simulink model "PI_current_no_modulatiob"  (R2018b)
settings: Solver=ode45  StartTime=0.0  StopTime=10  MaxStep=1e-3  RelTol=1e-6
values from neighbouring files (symbols this model uses):
  In = 189    [Motor_parameters_project.m]
  J = 0.0151    [Motor_parameters_project.m]
  Lm = 0.38e-3    (= 0.00038)    [Motor_parameters_project.m]
  Lr = Lm + Ldr    (= 0.00041116)    [Motor_parameters_project.m]
  Ls = Lm + Lds    (= 0.00041116)    [Motor_parameters_project.m]
  Omegae = 2*pi*fn    (= 364.424747816)    [Motor_parameters_project.m]
  p = 2.0    (= 2)    [Motor_parameters_project.m]
  Rr = 2.69e-3    (= 0.00269)    [Motor_parameters_project.m]
  Rs = 2.5e-3    (= 0.0025)    [Motor_parameters_project.m]
  Un = 24/sqrt(3)    [Motor_parameters_project.m]
undefined symbols (not defined in the file or in its folder): landa_r
settings Model: Creator=estef  LastModifiedBy=estef

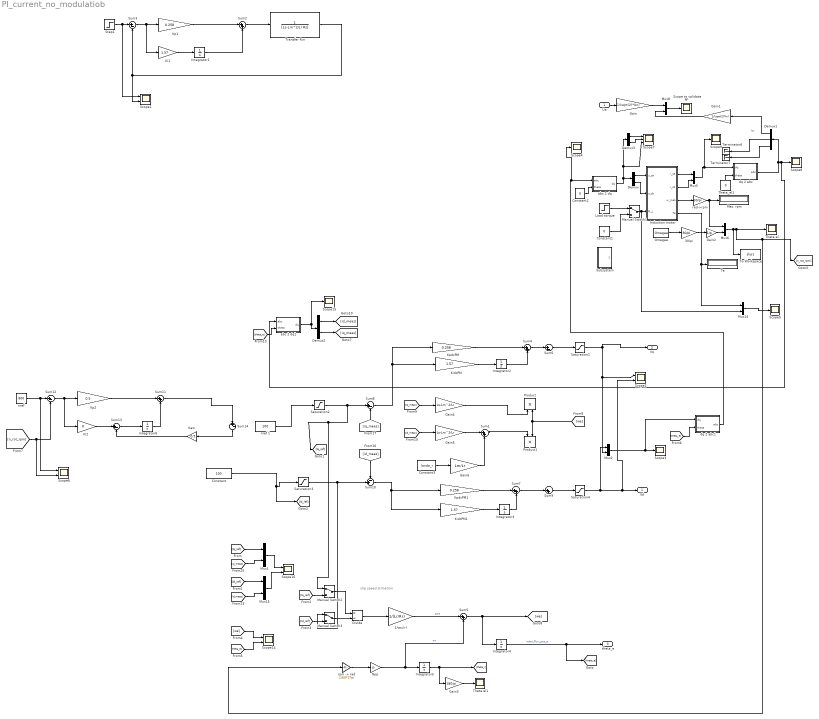
== system PI_current_no_modulatiob ==
  note: Ia
  note: slip speed stimation
  Ua : Inport
  1/tau(r) : Gain  Gain=1/(Lr/Rr)
  30/pi : Gain  Gain=30/pi
  Constant : Constant  Value=100
  Constant1 : Constant  Value=0
  Constant2 : Constant  Value=0
  Constant3 : Constant  Value=landa_r
  Demux : Demux  Outputs=2
  Demux1 : Demux  Outputs=3
  Demux2 : Demux  Outputs=2
  Demux3 : Demux  Outputs=2
  Divide : Product  Inputs=*/
  Gain : Gain  Gain=1/(sqrt(2)*Un)
  Gain1 : Gain  Gain=1/(sqrt(2)*In)
  Gain2 : Gain  Gain=1/p
  Gain3 : Gain  Gain=180/pi
  Gain4 : Gain  Gain=Ls-Lm^2/Lr
  Gain5 : Gain  Gain=Ls-Lm^2/Lr
  Gain6 : Gain  Gain=Lm/Lr
  Induction motor : Subsystem
  Integrator{1..6} (6 alike) : Integrator
  Kaw : Gain  Gain=0.5
  Ki1 : Gain  Gain=1.57
  Ki2 : Gain  Gain=0
  KidcPM : Gain  Gain=1.57
  KidcPM1 : Gain  Gain=1.57
  Kp1 : Gain  Gain=0.258
  Kp2 : Gain  Gain=0.5
  KpdcPM : Gain  Gain=0.258
  KpdcPM1 : Gain  Gain=0.258
  Load torque : Step  Time=0.9  After=5  SampleTime=0
  Manual Switch1 : ManualSwitch
  Manual Switch2 : ManualSwitch
  Manual Switch3 : ManualSwitch
  Mec. rpm : Display
  Mux{1..2,5..6,8,14..15} (7 alike) : Mux  Inputs=2
  Npp : Gain  Gain=p  SaturateOnIntegerOverflow=on  OutDataTypeStr=Inherit: Same as input  ParamDataTypeStr=Inherit: Same as input
  Omegae : Constant  Value=Omegae
  Product : Product  SaturateOnIntegerOverflow=on  InputSameDT=on  OutDataTypeStr=Inherit: Same as first input
  Product1 : Product  SaturateOnIntegerOverflow=on  InputSameDT=on  OutDataTypeStr=Inherit: Same as first input
  Saturation1 : Saturate  UpperLimit=Un*sqrt(2)  LowerLimit=-Un*sqrt(2)
  Saturation2 : Saturate  UpperLimit=In*sqrt(2)  LowerLimit=-In*sqrt(2)
  Saturation3 : Saturate  UpperLimit=In*sqrt(2)  LowerLimit=-In*sqrt(2)
  Saturation4 : Saturate  UpperLimit=Un*sqrt(2)  LowerLimit=-Un*sqrt(2)
  Scope to validate PF : Scope
  Scope{1..2,6,14,16} (5 alike) : Scope  NumInputPorts=2
  Scope{3..5,8..9,15} (6 alike) : Scope
  Scope7 : Scope  NumInputPorts=3
  Step1 : Step  Time=0.1  After=100  SampleTime=0
  Subsystem : Subsystem
  Sum{1..2,4..5,7,9,11} (7 alike) : Sum  Inputs=|++
  Sum10 : Sum  Inputs=-+|  SaturateOnIntegerOverflow=on  InputSameDT=on  OutDataTypeStr=Inherit: Same as first input
  Sum{3,6,12..14} (5 alike) : Sum  Inputs=|+-
  Sum8 : Sum  Inputs=|+-  SaturateOnIntegerOverflow=on  InputSameDT=on  OutDataTypeStr=Inherit: Same as first input
  Te : Display
  Terminator6 : Terminator
  Terminator7 : Terminator
  Theta.el : Scope
  Theta.el1 : Scope
  Theta_el1 : Constant  Value=0
  To Workspace : ToWorkspace  VariableName=slip1  SaveFormat=Timeseries  SampleTime=-1
  Transfer Fcn : TransferFcn  Denominator=[Ls-Lm^2/Lr Rs]
  abc 2 dq : Subsystem
  abc 2 dq1 : Subsystem
  dq 2 abc : Subsystem
  dq 2 abc1 : Subsystem
  "nref " : Constant  Value=800
  nref 1 : Constant  Value=100
  rad->rpm : Gain  Gain=30/pi  SaturateOnIntegerOverflow=on  OutDataTypeStr=Inherit: Same as input  ParamDataTypeStr=Inherit: Same as input
  "rpm -> rad" : Gain  Gain=1/60*2*pi  SaturateOnIntegerOverflow=on  OutDataTypeStr=Inherit: Same as input  ParamDataTypeStr=Inherit: Same as input
  Vd : Outport
  "Vq " : Outport  Port=2
  "theta_e " : Outport  Port=3
  wires:
  Ki1/1 -> Integrator1/1
  Sum3/1 -> Ki1/1, Kp1/1
  Step1/1 -> Scope1/1, Sum3/1
  Kp1/1 -> Sum2/1
  Integrator1/1 -> Sum2/2
  Transfer Fcn/1 -> Sum3/2, Scope1/2
  Mux5/1 -> Scope9/1, dq 2 abc/1(dq)
  abc 2 dq/1(dq) -> Scope7/3, Demux3/1, Demux/1
  Induction motor/1(i_sa) -> Mux5/1
  30/pi/1 -> Gain2/1
  Demux3/1 -> Scope7/1
  Induction motor/3(w_mek) -> rad->rpm/1
  Demux1/1 -> Gain1/1
  Demux/1 -> Induction motor/1(u_sa)
  Load torque/1 -> Manual Switch1/1
  Mux14/1 -> Scope5/1
  Theta_el1/1 -> dq 2 abc/2(theta)
  Induction motor/2(i_sb) -> Mux5/2
  Omegae/1 -> 30/pi/1
  Demux3/2 -> Scope7/2
  Gain2/1 -> Mux6/2
  Gain1/1 -> Mux8/2
  Induction motor/4(Te) -> Mux14/1, Te/1
  Manual Switch1/1 -> Mux14/2, Induction motor/3(M_L)
  Demux1/3 -> Terminator7/1
  Mux8/1 -> Scope to validate PF/1
  Demux1/2 -> Terminator6/1
  rad->rpm/1 -> Mux6/1, Mec. rpm/1
  Gain/1 -> Mux8/1
  Ua/1 -> Gain/1
  Demux/2 -> Induction motor/2(u_sb)
  Constant2/1 -> abc 2 dq/2(theta)
  Integrator3/1 -> Sum7/2
  KidcPM1/1 -> Integrator3/1
  KidcPM/1 -> Integrator2/1
  Manual Switch2/1 -> Divide/1
  [Id_ref] -> Manual Switch3/2
  Manual Switch3/1 -> Divide/2
  Saturation3/1 -> Manual Switch3/1, Sum10/2
  dq 2 abc/1(abc) -> Demux1/1, abc 2 dq1/1(abc), Scope8/1
  [iq_meas] -> Sum8/2
  KpdcPM/1 -> Sum4/1
  Divide/1 -> 1/tau(r)/1
  Mux15/1 -> Scope16/2
  Saturation2/1 -> Manual Switch2/1, [Iq_ref], Sum8/1
  Sum10/1 -> KidcPM1/1, KpdcPM1/1
  [Id_ref] -> Mux15/1
  Npp/1 -> Integrator5/1, Sum5/2  "wr"
  Gain3/1 -> Theta.el1/1
  abc 2 dq1/1(dq) -> Demux2/1, Scope15/1
  "rpm -> rad"/1 -> Npp/1
  Sum8/1 -> KidcPM/1, KpdcPM/1
  Demux2/2 -> [iq_meas]
  KpdcPM1/1 -> Sum7/1
  [id_meas] -> Mux15/2
  Mux2/1 -> dq 2 abc1/1(dq), Scope3/1
  Integrator5/1 -> [theta_r], Gain3/1
  Integrator2/1 -> Sum4/2
  [we] -> Scope14/1
  [theta_e] -> Scope14/2
  [id_meas] -> Sum10/1
  Demux2/1 -> [id_meas]
  [theta_e] -> abc 2 dq1/2(theta)
  [Iq_ref] -> Manual Switch2/2
  Mux6/1 -> To Workspace/1, "rpm -> rad"/1, [n_rot_rpm], Theta.el/1
  [Iq_ref] -> Mux1/1
  1/tau(r)/1 -> Sum5/1  "swe"
  Mux1/1 -> Scope16/1
  Sum5/1 -> Integrator4/1, [we]
  [iq_meas] -> Mux1/2
  Integrator4/1 -> [theta_e], "theta_e "/1  "rotor_flux_pos_e"
  [theta_e] -> dq 2 abc1/2(theta)
  dq 2 abc1/1(abc) -> Scope4/1, abc 2 dq/1(abc)
  Saturation1/1 -> "Vq "/1, Mux2/2, Scope2/1
  Saturation4/1 -> Mux2/1, Scope2/2, Vd/1
  Constant/1 -> [Id_ref], Saturation3/1
  Sum12/1 -> Ki2/1, Kp2/1
  Integrator6/1 -> Sum11/2
  "nref "/1 -> Scope6/1, Sum12/1
  Kp2/1 -> Sum11/1
  [n_rot_rpm] -> Scope6/2, Sum12/2
  Ki2/1 -> Sum13/1
  Sum13/1 -> Integrator6/1
  Sum11/1 -> Sum14/1
  Sum14/1 -> Kaw/1
  Kaw/1 -> Sum13/2
  nref 1/1 -> Saturation2/1
  Constant1/1 -> Manual Switch1/2
  Sum2/1 -> Transfer Fcn/1
  [id_meas] -> Gain5/1
  Gain5/1 -> Sum1/1
  [iq_meas] -> Gain4/1
  Gain6/1 -> Sum1/2
  [we] -> Product1/2, Product/2
  Gain4/1 -> Product/1
  Constant3/1 -> Gain6/1
  Sum1/1 -> Product1/1
  Sum4/1 -> Sum6/1
  Sum6/1 -> Saturation1/1
  Sum7/1 -> Sum9/1
  Sum9/1 -> Saturation4/1

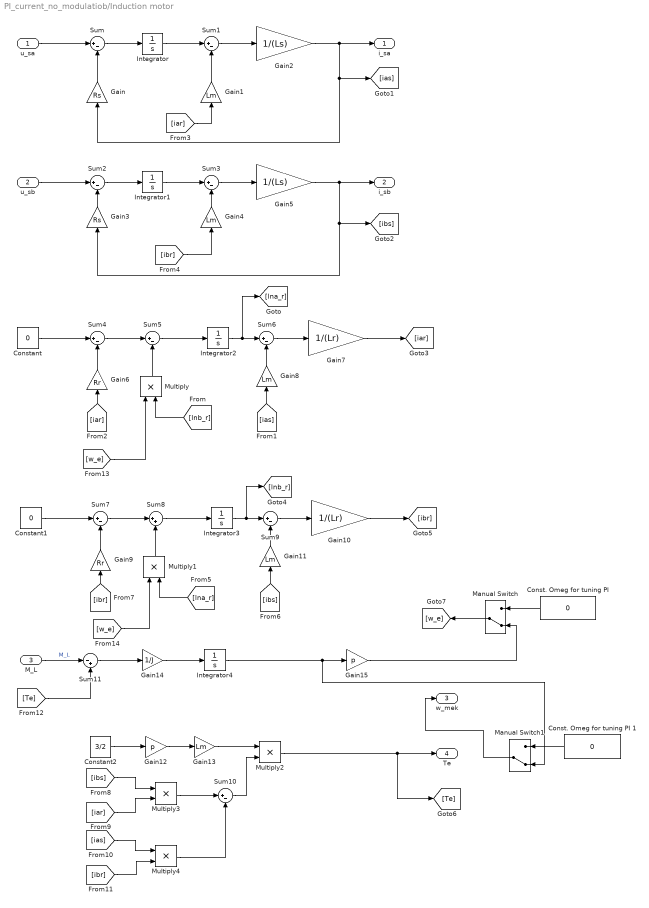
== system PI_current_no_modulatiob/Induction motor ==
  u_sa : Inport
  u_sb : Inport  Port=2
  M_L : Inport  Port=3
  "Const. Omeg for tuning PI " : Constant  Value=0
  Const. Omeg for tuning PI 1 : Constant  Value=0
  Constant : Constant  Value=0
  Constant1 : Constant  Value=0
  Constant2 : Constant  Value=3/2
  Gain : Gain  Gain=Rs
  Gain{1,4,8,11,13} (5 alike) : Gain  Gain=Lm
  Gain10 : Gain  Gain=1/(Lr)
  Gain12 : Gain  Gain=p
  Gain14 : Gain  Gain=1/J
  Gain15 : Gain  Gain=p
  Gain2 : Gain  Gain=1/(Ls)
  Gain3 : Gain  Gain=Rs
  Gain5 : Gain  Gain=1/(Ls)
  Gain6 : Gain  Gain=Rr
  Gain7 : Gain  Gain=1/(Lr)
  Gain9 : Gain  Gain=Rr
  Integrator{,1..4} (5 alike) : Integrator
  Manual Switch : ManualSwitch  CurrentSetting=0
  Manual Switch1 : ManualSwitch  CurrentSetting=0
  Multiply{,1..4} (5 alike) : Product
  Sum{,1..7,9..10} (10 alike) : Sum  Inputs=|+-
  Sum11 : Sum  Inputs=|-+
  Sum8 : Sum  Inputs=|++
  i_sa : Outport
  i_sb : Outport  Port=2
  w_mek : Outport  Port=3
  Te : Outport  Port=4
  wires:
  u_sa/1 -> Sum/1
  Gain/1 -> Sum/2
  Sum/1 -> Integrator/1
  Integrator/1 -> Sum1/1
  Gain1/1 -> Sum1/2
  Sum1/1 -> Gain2/1
  Gain2/1 -> [ias], Gain/1, i_sa/1
  Gain3/1 -> Sum2/2
  u_sb/1 -> Sum2/1
  Sum3/1 -> Gain5/1
  Gain4/1 -> Sum3/2
  Gain5/1 -> i_sb/1, [ibs], Gain3/1
  Sum2/1 -> Integrator1/1
  Integrator1/1 -> Sum3/1
  Constant/1 -> Sum4/1
  Gain6/1 -> Sum4/2
  Sum4/1 -> Sum5/1
  [lnb_r] -> Multiply/2
  Sum5/1 -> Integrator2/1
  Gain8/1 -> Sum6/2
  [ias] -> Gain8/1
  Integrator2/1 -> [lna_r], Sum6/1
  Sum6/1 -> Gain7/1
  Multiply/1 -> Sum5/2
  Gain7/1 -> [iar]
  [iar] -> Gain6/1
  [ibr] -> Gain4/1
  [iar] -> Gain1/1
  Gain11/1 -> Sum9/2
  Gain10/1 -> [ibr]
  [ibr] -> Gain9/1
  [ibs] -> Gain11/1
  Multiply1/1 -> Sum8/2
  Integrator3/1 -> [lnb_r], Sum9/1
  Sum7/1 -> Sum8/1
  [lna_r] -> Multiply1/2
  Gain9/1 -> Sum7/2
  Sum9/1 -> Gain10/1
  Sum8/1 -> Integrator3/1
  Constant1/1 -> Sum7/1
  Gain13/1 -> Multiply2/1
  Sum10/1 -> Multiply2/2
  [ibs] -> Multiply3/1
  [iar] -> Multiply3/2
  Multiply3/1 -> Sum10/1
  [ias] -> Multiply4/1
  [ibr] -> Multiply4/2
  Multiply4/1 -> Sum10/2
  Constant2/1 -> Gain12/1
  Gain12/1 -> Gain13/1
  Multiply2/1 -> [Te], Te/1
  [Te] -> Sum11/2
  M_L/1 -> Sum11/1  "M_L"
  Sum11/1 -> Gain14/1
  Gain14/1 -> Integrator4/1
  Integrator4/1 -> Manual Switch1/2, Gain15/1
  [w_e] -> Multiply/1
  [w_e] -> Multiply1/1
  "Const. Omeg for tuning PI "/1 -> Manual Switch/1
  Gain15/1 -> Manual Switch/2
  Manual Switch/1 -> [w_e]
  Const. Omeg for tuning PI 1/1 -> Manual Switch1/1
  Manual Switch1/1 -> w_mek/1

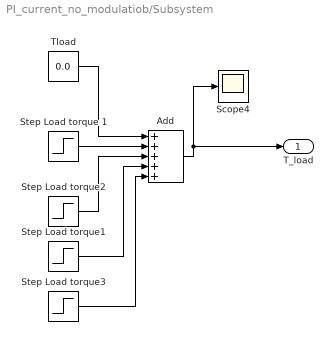
== system PI_current_no_modulatiob/Subsystem ==
  Add : Sum  Inputs=+++++
  Scope4 : Scope
  Step Load torque 1 : Step  Time=0.9  After=5  SampleTime=0
  Step Load torque1 : Step  Time=5  After=8  SampleTime=0
  Step Load torque2 : Step  Time=3  After=8  SampleTime=0
  Step Load torque3 : Step  Time=7  After=10  SampleTime=0
  Tload : Constant  Value=0.0
  T_load : Outport
  wires:
  Add/1 -> T_load/1, Scope4/1
  Step Load torque 1/1 -> Add/2
  Tload/1 -> Add/1
  Step Load torque2/1 -> Add/3
  Step Load torque1/1 -> Add/4
  Step Load torque3/1 -> Add/5

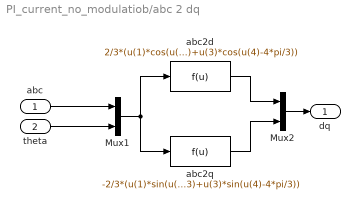
== system PI_current_no_modulatiob/abc 2 dq ==
  abc : Inport
  theta : Inport  Port=2
  Mux1 : Mux  Inputs=2
  Mux2 : Mux  Inputs=2
  abc2d : Fcn  Expr=2/3*(u(1)*cos(u(4))+u(2)*cos(u(4)-2*pi/3)+u(3)*cos(u(4)-4*pi/3))
  abc2q : Fcn  Expr=-2/3*(u(1)*sin(u(4))+u(2)*sin(u(4)-2*pi/3)+u(3)*sin(u(4)-4*pi/3))
  dq : Outport
  wires:
  abc/1 -> Mux1/1
  theta/1 -> Mux1/2
  Mux1/1 -> abc2d/1, abc2q/1
  abc2d/1 -> Mux2/1
  abc2q/1 -> Mux2/2
  Mux2/1 -> dq/1

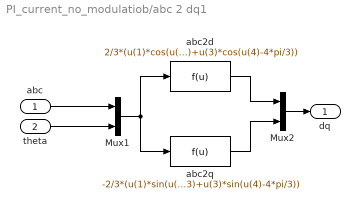
== system PI_current_no_modulatiob/abc 2 dq1 ==
  abc : Inport
  theta : Inport  Port=2
  Mux1 : Mux  Inputs=2
  Mux2 : Mux  Inputs=2
  abc2d : Fcn  Expr=2/3*(u(1)*cos(u(4))+u(2)*cos(u(4)-2*pi/3)+u(3)*cos(u(4)-4*pi/3))
  abc2q : Fcn  Expr=-2/3*(u(1)*sin(u(4))+u(2)*sin(u(4)-2*pi/3)+u(3)*sin(u(4)-4*pi/3))
  dq : Outport
  wires:
  abc/1 -> Mux1/1
  theta/1 -> Mux1/2
  Mux1/1 -> abc2d/1, abc2q/1
  abc2d/1 -> Mux2/1
  abc2q/1 -> Mux2/2
  Mux2/1 -> dq/1

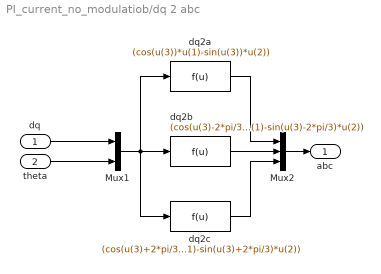
== system PI_current_no_modulatiob/dq 2 abc ==
  dq : Inport
  theta : Inport  Port=2
  Mux1 : Mux  Inputs=2
  Mux2 : Mux  Inputs=3
  dq2a : Fcn  Expr=(cos(u(3))*u(1)-sin(u(3))*u(2))
  dq2b : Fcn  Expr=(cos(u(3)-2*pi/3)*u(1)-sin(u(3)-2*pi/3)*u(2))
  dq2c : Fcn  Expr=(cos(u(3)+2*pi/3)*u(1)-sin(u(3)+2*pi/3)*u(2))
  abc : Outport
  wires:
  Mux2/1 -> abc/1
  dq2b/1 -> Mux2/2
  dq2a/1 -> Mux2/1
  Mux1/1 -> dq2a/1, dq2c/1, dq2b/1
  theta/1 -> Mux1/2
  dq/1 -> Mux1/1
  dq2c/1 -> Mux2/3

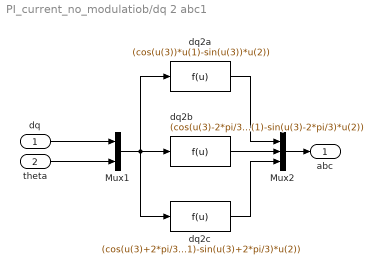
== system PI_current_no_modulatiob/dq 2 abc1 ==
  dq : Inport
  theta : Inport  Port=2
  Mux1 : Mux  Inputs=2
  Mux2 : Mux  Inputs=3
  dq2a : Fcn  Expr=(cos(u(3))*u(1)-sin(u(3))*u(2))
  dq2b : Fcn  Expr=(cos(u(3)-2*pi/3)*u(1)-sin(u(3)-2*pi/3)*u(2))
  dq2c : Fcn  Expr=(cos(u(3)+2*pi/3)*u(1)-sin(u(3)+2*pi/3)*u(2))
  abc : Outport
  wires:
  Mux2/1 -> abc/1
  dq2b/1 -> Mux2/2
  dq2a/1 -> Mux2/1
  Mux1/1 -> dq2a/1, dq2c/1, dq2b/1
  theta/1 -> Mux1/2
  dq/1 -> Mux1/1
  dq2c/1 -> Mux2/3
